simulink library "subsystems"  (R2025b)
settings: Solver=VariableStepAuto  StartTime=0.0  StopTime=10.0  RelTol=1e-3
values from neighbouring files (symbols this model uses):
  Cmdot = 1.2827224    [plant_parameters.m]
  cv = 718    [plant_parameters.m]
  g = [0 0 -9.80665]    [plant_parameters.m]
  m0 = 3.1359    [plant_parameters.m]
  T0 = 300    [plant_parameters.m]
  tank_volume = 0.009    [plant_parameters.m]
undefined symbols (not defined in the file or in its folder): DiscIntNeverNeededParam, force_controller_Ts, motor, Nozzle, platform_vel_controller, position_controller, position_controller_Ts, pressure_controller, velocity_controller, velocity_controller_Ts
libraries: simulink x14, $bdroot x6, spsFirstOrderFilterLib x2, slident x1, eeGeneralControl x1
settings Model: Creator=karadeli  LastModifiedBy=karadeli

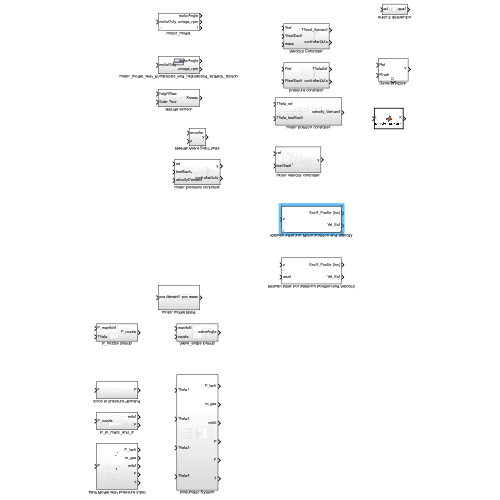
[thumbnail: Simulink's stored preview of the top-level diagram]
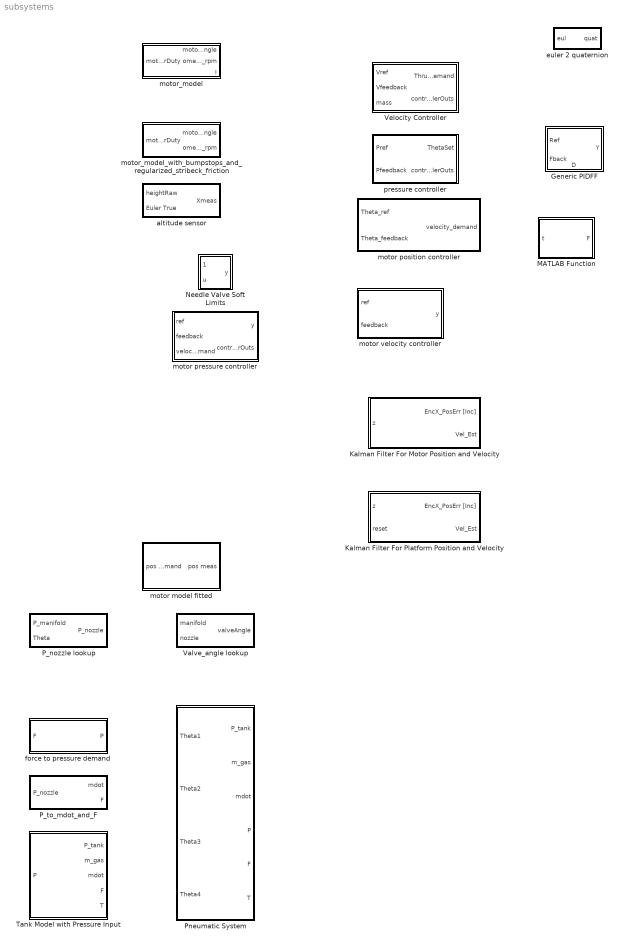
== system subsystems ==
  Generic PIDFF : Subsystem  mask{kP=0, kI=0, kD=0, kFF=0, saturation=0, saturationInt=0, rateLim=0, inputSat=0, derivativeTimeConst=0, Ts=1e-3}
      settings: PortSchema="{\"entries\":[{\"content\":{\"sides\":[{\"content\":{\"connectorIds\":[\"In1\",\"In2\"]},\"type\":\"ConnectorPlacement.EquallySpacedRectSide\",\"uuid\":\"19262ba2-78ba-44a2-8781-9b98a158f546\"},{\"content\":{\"connectorIds\":[\"Out1\"],\"side\":\"RIGHT\"},\"type\":\"ConnectorPlacement.EquallySpacedRectSide\",\"uuid\":\"f142a127-8a5f-4ee4-b1f0-7b86e0ffd133\"},{\"content\":{\"side\":\"TOP\"},\"type\":\"ConnectorPlacement.EquallySpacedRectSide\",\"uuid\":\"38fd1d3f-0c0d-4b7a-8dea-b06c7855f656\"},{\"content\":{\"connectorIds\":[\"Out2\"],\"side\":\"BOTTOM\"},\"type\":\"ConnectorPlacement.EquallySpacedRectSide\",\"uuid\":\"c6a4933e-73d5-49a0-b95d-1775e13b11db\"}]},\"type\":\"ConnectorPlacement.EquallySpacedConnector\",\"uuid\":\"e308508e-a04b-47c8-be17-ad9ebf164901\"}],\"packageUris\":[\"http://schema.mathworks.com/mf0/Connector/R2020b\"],\"version\":\"1.0\"}"
  Kalman Filter For Motor Position and Velocity : Subsystem  mask{Ts=1e-3, lambda_RQ=1}
      mask prompts: Ts "Tsample (s)"
  Kalman Filter For Platform Position and Velocity : Subsystem  mask{Ts=1e-3}
      mask prompts: Ts "Tsample (s)"
  MATLAB Function : MATLAB Function  TreatAsAtomicUnit=on
  Needle Valve Soft Limits : Subsystem
  P_nozzle lookup : Subsystem
  P_to_mdot_and_F : Subsystem
  Pneumatic System : Subsystem
  Tank Model with Pressure Input : Subsystem
  Valve_angle lookup : Subsystem
  Velocity Controller : Subsystem
  altitude sensor : Subsystem
  euler 2 quaternion : Subsystem
  force to pressure demand : Subsystem
  motor model fitted : Subsystem
  motor position controller : Subsystem
  motor pressure controller : Subsystem
  motor velocity controller : Subsystem
  motor_model : Subsystem  AncestorBlock=subsystems/motor_model_with_bumpstops_and_regularized_stribeck_friction  mask{R=6.17, Km=3.1e-2, bv=1e-4, J=1e-5, Vn=24, L=1e-6}
  motor_model_with_bumpstops_and_regularized_stribeck_friction : Subsystem
  pressure controller : Subsystem

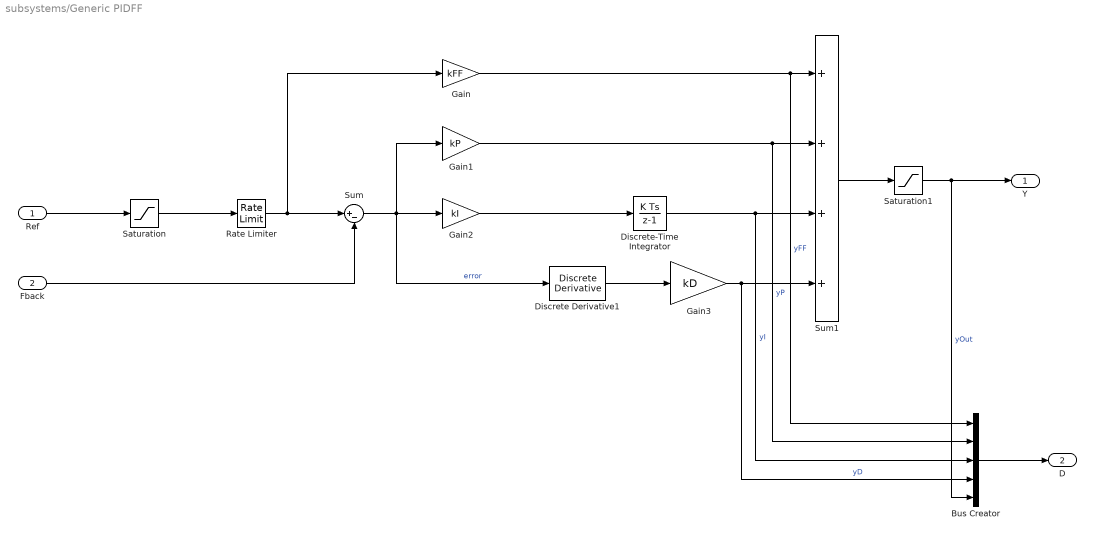
== system subsystems/Generic PIDFF ==
  Ref : Inport  PortDimensions=1  SampleTime=Ts
  Fback : Inport  Port=2  PortDimensions=1  SampleTime=Ts
  Bus Creator : BusCreator  Inputs=5
  Discrete Derivative1 : simulink/Discrete/Discrete Derivative  gainval=1.0  ICPrevScaledInput=0.0  OutMin=[]  OutMax=[]  OutDataType=fixdt(1, 16)  OutScaling=2^-10  DoSatur=off
  Discrete-Time Integrator : DiscreteIntegrator  SampleTime=Ts  LimitOutput=on  UpperSaturationLimit=saturationInt  LowerSaturationLimit=-saturationInt  ICPrevOutput=DiscIntNeverNeededParam  ICPrevScaledInput=DiscIntNeverNeededParam
  Gain : Gain  Gain=kFF
  Gain1 : Gain  Gain=kP
  Gain2 : Gain  Gain=kI
  Gain3 : Gain  Gain=kD
  Rate Limiter : RateLimiter  RisingSlewLimit=rateLim  FallingSlewLimit=-rateLim  SampleTimeMode=inherited
  Saturation : Saturate  UpperLimit=inputSat  LowerLimit=-inputSat
  Saturation1 : Saturate  UpperLimit=saturation  LowerLimit=-saturation
  Sum : Sum  Inputs=|+-
  Sum1 : Sum  Inputs=++++
  Y : Outport  PortDimensions=1  SampleTime=Ts
  D : Outport  Port=2  SampleTime=Ts
  wires:
  Bus Creator/1 -> D/1
  Discrete-Time Integrator/1 -> Sum1/3, Bus Creator/3  "yI"
  Gain1/1 -> Sum1/2, Bus Creator/2  "yP"
  Gain3/1 -> Sum1/4, Bus Creator/4  "yD"
  Saturation1/1 -> Bus Creator/5, Y/1  "yOut"
  Gain/1 -> Sum1/1, Bus Creator/1  "yFF"
  Fback/1 -> Sum/2
  Ref/1 -> Saturation/1
  Rate Limiter/1 -> Sum/1, Gain/1
  Saturation/1 -> Rate Limiter/1
  Sum/1 -> Discrete Derivative1/1, Gain2/1, Gain1/1  "error"
  Gain2/1 -> Discrete-Time Integrator/1
  Sum1/1 -> Saturation1/1
  Discrete Derivative1/1 -> Gain3/1

== system subsystems/Kalman Filter For Motor Position and Velocity ==
  z : Inport  Unit=deg  PortDimensions=1
  Resettable Delay_qk : Delay  DelayLength=1  InitialConditionSource=Input port  SampleTime=Ts
      settings: InputPortMap=u0,p4
  TPE_KALMAN_spd : MATLAB Function  TreatAsAtomicUnit=on
  Unit Delay_Pk : UnitDelay  InitialCondition=[0.155 65; 65 5.7e4]  SampleTime=Ts  HasFrameUpgradeWarning=on
  lambda_RQ : Constant  Value=lambda_RQ  OutDataTypeStr=double
  EncX_PosErr [Inc] : Outport  OutDataTypeStr=double  Unit=deg  PortDimensions=1  SampleTime=Ts  VectorParamsAs1DForOutWhenUnconnected=off
  Vel_Est : Outport  Port=2  OutDataTypeStr=double  Unit=deg/s  PortDimensions=1  SampleTime=Ts  VectorParamsAs1DForOutWhenUnconnected=off
  wires:
  Unit Delay_Pk/1 -> TPE_KALMAN_spd/4("Pk ")
  TPE_KALMAN_spd/2(posEst) -> EncX_PosErr [Inc]/1  "Pos_Est"
  Resettable Delay_qk/1 -> TPE_KALMAN_spd/3("qk ")
  TPE_KALMAN_spd/4(Pk) -> Unit Delay_Pk/1
  TPE_KALMAN_spd/3(qk) -> Resettable Delay_qk/1  "qk"
  z/1 -> Resettable Delay_qk/2, TPE_KALMAN_spd/2(z)
  lambda_RQ/1 -> TPE_KALMAN_spd/1(lambdaRQ)
  TPE_KALMAN_spd/1(velEst) -> Vel_Est/1  "Vel_Est"

== system subsystems/Kalman Filter For Platform Position and Velocity ==
  z : Inport  Unit=m  PortDimensions=1
  reset : Inport  Port=2  PortDimensions=1
  MATLAB Function : MATLAB Function  TreatAsAtomicUnit=on
  Resettable Delay_qk : Delay  DelayLength=1  InitialConditionSource=Input port  ExternalReset=Rising  SampleTime=Ts
      settings: InputPortMap=u0,r5,p4
  TPE_KALMAN_spd : MATLAB Function  TreatAsAtomicUnit=on
  Unit Delay_Pk : UnitDelay  InitialCondition=[0.155 65; 65 5.7e4]  SampleTime=Ts  HasFrameUpgradeWarning=on
  lambda_RQ : Constant  Value=2e-5  OutDataTypeStr=double
  z1 : InportShadow  Unit=m  PortDimensions=1
  EncX_PosErr [Inc] : Outport  OutDataTypeStr=double  Unit=m  PortDimensions=1  SampleTime=Ts  VectorParamsAs1DForOutWhenUnconnected=off
  Vel_Est : Outport  Port=2  OutDataTypeStr=double  Unit=m/s  PortDimensions=1  SampleTime=Ts  VectorParamsAs1DForOutWhenUnconnected=off
  wires:
  TPE_KALMAN_spd/1(velEst) -> Vel_Est/1  "Vel_Est"
  lambda_RQ/1 -> TPE_KALMAN_spd/1(lambdaRQ)
  z/1 -> TPE_KALMAN_spd/2(z)
  TPE_KALMAN_spd/3(qk) -> Resettable Delay_qk/1  "qk"
  TPE_KALMAN_spd/4(Pk) -> Unit Delay_Pk/1
  Resettable Delay_qk/1 -> TPE_KALMAN_spd/3("qk ")
  TPE_KALMAN_spd/2(posEst) -> EncX_PosErr [Inc]/1  "Pos_Est"
  Unit Delay_Pk/1 -> TPE_KALMAN_spd/4("Pk ")
  MATLAB Function/1(y) -> Resettable Delay_qk/3
  z1/1 -> MATLAB Function/1(u1)
  reset/1 -> Resettable Delay_qk/2

== system subsystems/Needle Valve Soft Limits ==
  encoder : Inport
  u : Inport  Port=2
  Constant1 : Constant  Value=-1
  Constant2 : Constant  Value=0
  Constant3 : Constant
  Constant4 : Constant  Value=0
  Saturation Dynamic : simulink/Discontinuities/Saturation Dynamic  OutMin=[]  OutMax=[]  OutDataTypeStr=Inherit: Same as second input  OutDataType=fixdt(1, 16)  OutScaling=2^-10  DoSatur=off
  Switch : Switch  Criteria=u2 > Threshold  Threshold=3*360  SaturateOnIntegerOverflow=off  InputSameDT=off
  Switch1 : Switch  Criteria=u2 > Threshold  Threshold=10  SaturateOnIntegerOverflow=off  InputSameDT=off
  y : Outport
  wires:
  Constant1/1 -> Switch1/1
  Constant4/1 -> Switch1/3
  u/1 -> Saturation Dynamic/2
  Switch1/1 -> Saturation Dynamic/3
  encoder/1 -> Switch/2, Switch1/2
  Constant3/1 -> Switch/3
  Constant2/1 -> Switch/1
  Switch/1 -> Saturation Dynamic/1
  Saturation Dynamic/1 -> y/1

== system subsystems/P_nozzle lookup ==
  P_manifold : Inport
  Theta : Inport  Port=2
  P_nozzle lookup : MATLAB Function  Commented=on  TreatAsAtomicUnit=on
  P_nozzle lookup1 : MATLAB Function  TreatAsAtomicUnit=on
  Saturation : Saturate  UpperLimit=300  LowerLimit=0
  P_nozzle : Outport
  wires:
  P_manifold/1 -> P_nozzle lookup1/1(manifold)
  Theta/1 -> P_nozzle lookup1/2(valveAngle)
  P_nozzle lookup1/1(nozzlePressure) -> Saturation/1
  Saturation/1 -> P_nozzle/1

== system subsystems/P_to_mdot_and_F ==
  P_nozzle : Inport  Unit=bar
  Gain : Gain  Gain=Nozzle.Cd
  Gain1 : Gain  Gain=1e5
  Ve1 : Gain  Gain=Nozzle.M * sqrt(1.4 * 287 / (1 + (0.2 .* Nozzle.M .* Nozzle.M)) * 300)
  kMdot3 : Gain  Gain="0.6847*pi*(Nozzle.d  * Nozzle.d)/4*1e-6/sqrt(287*300)"
  mdot : Outport  Unit=kg/s
  F : Outport  Port=2  Unit=N
  wires:
  P_nozzle/1 -> Gain1/1  "Bar"
  kMdot3/1 -> Ve1/1, mdot/1  "mdot"
  Ve1/1 -> Gain/1  "Ftheoretical"
  Gain/1 -> F/1  "Factual"
  Gain1/1 -> kMdot3/1  "Pa"

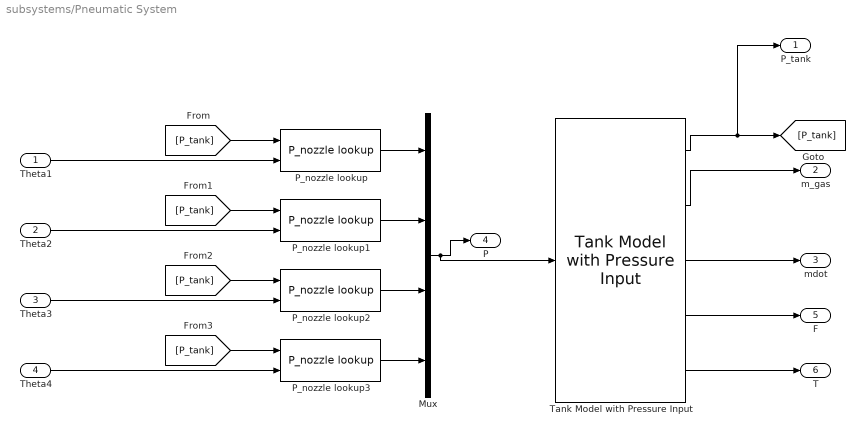
== system subsystems/Pneumatic System ==
  Theta1 : Inport
  Theta2 : Inport  Port=2
  Theta3 : Inport  Port=3
  Theta4 : Inport  Port=4
  Mux : Mux
  P_nozzle lookup{,1..3} (4 alike) : $bdroot/P_nozzle lookup  SystemSampleTime=-1  VariantActivationTime=update diagram  EmptyChoice=off  PassThrough=off  PassThroughVariantControl=(default)  EmptyChoiceVariantControl=(default)  AllowFlexibleInterface=on  Latency=0  AutoFrameSizeCalculation=off
  Tank Model with Pressure Input : $bdroot/Tank Model with Pressure Input  SystemSampleTime=-1  VariantActivationTime=update diagram  EmptyChoice=off  PassThrough=off  PassThroughVariantControl=(default)  EmptyChoiceVariantControl=(default)  AllowFlexibleInterface=on  Latency=0  AutoFrameSizeCalculation=off
  P_tank : Outport
  m_gas : Outport  Port=2
  mdot : Outport  Port=3
  P : Outport  Port=4
  F : Outport  Port=5
  T : Outport  Port=6
  wires:
  Tank Model with Pressure Input/1 -> P_tank/1, [P_tank]
  [P_tank] -> P_nozzle lookup/1
  Theta1/1 -> P_nozzle lookup/2
  Tank Model with Pressure Input/2 -> m_gas/1
  Tank Model with Pressure Input/3 -> mdot/1
  Tank Model with Pressure Input/4 -> F/1
  Tank Model with Pressure Input/5 -> T/1
  P_nozzle lookup/1 -> Mux/1
  Theta2/1 -> P_nozzle lookup1/2
  [P_tank] -> P_nozzle lookup1/1
  [P_tank] -> P_nozzle lookup3/1
  Theta4/1 -> P_nozzle lookup3/2
  Theta3/1 -> P_nozzle lookup2/2
  [P_tank] -> P_nozzle lookup2/1
  P_nozzle lookup3/1 -> Mux/4
  P_nozzle lookup2/1 -> Mux/3
  P_nozzle lookup1/1 -> Mux/2
  Mux/1 -> Tank Model with Pressure Input/1, P/1

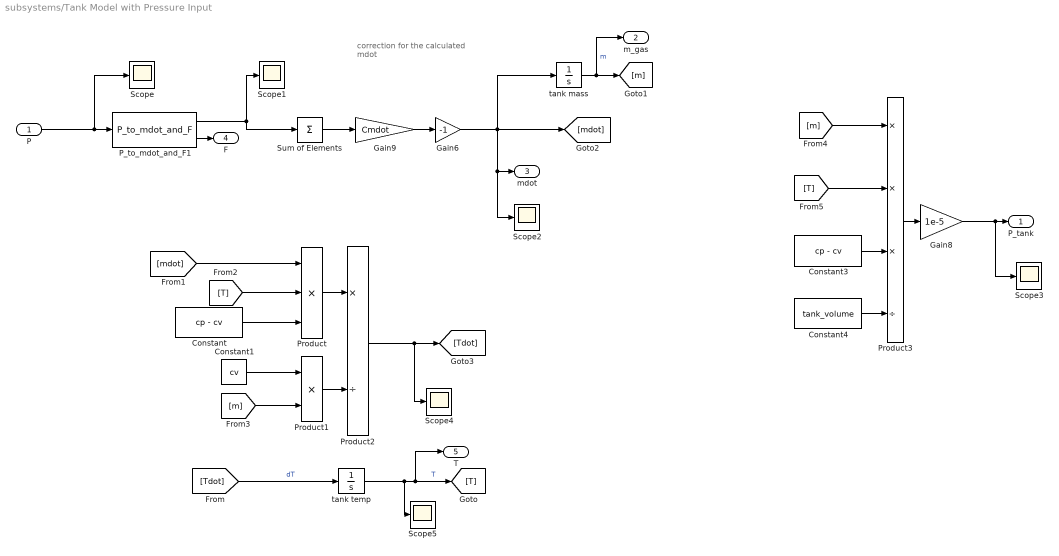
== system subsystems/Tank Model with Pressure Input ==
  note: correction for the calculated mdot
  P : Inport
  Constant : Constant  Value=cp - cv
  Constant1 : Constant  Value=cv
  Constant3 : Constant  Value=cp - cv
  Constant4 : Constant  Value=tank_volume
  Gain6 : Gain  Gain=-1
  Gain8 : Gain  Gain=1e-5
  Gain9 : Gain  Gain=Cmdot
  P_to_mdot_and_F1 : $bdroot/P_to_mdot_and_F  SystemSampleTime=-1  VariantActivationTime=update diagram  AllowFlexibleInterface=on  Latency=0  AutoFrameSizeCalculation=off
  Product : Product  Inputs=3
  Product1 : Product
  Product2 : Product  Inputs=*/
  Product3 : Product  Inputs=***/
  Scope{,1..5} (6 alike) : Scope
      Scope1 settings: DataLoggingVariableName=ScopeData2
      Scope2 settings: DataLoggingVariableName=ScopeData3
      Scope3 settings: DataLoggingVariableName=ScopeData4
      Scope4 settings: DataLoggingVariableName=ScopeData5
      Scope5 settings: DataLoggingVariableName=ScopeData6
  Sum of Elements : Sum  Inputs=+
  tank mass : Integrator  InitialCondition=m0  LimitOutput=on  LowerSaturationLimit=0
  tank temp : Integrator  InitialCondition=T0
  P_tank : Outport
  m_gas : Outport  Port=2
  mdot : Outport  Port=3
  F : Outport  Port=4
  T : Outport  Port=5
  wires:
  Constant3/1 -> Product3/3
  [T] -> Product/2
  tank mass/1 -> m_gas/1, [m]  "m"
  Gain9/1 -> Gain6/1
  [m] -> Product3/1
  Sum of Elements/1 -> Gain9/1
  [Tdot] -> tank temp/1  "dT"
  Product3/1 -> Gain8/1
  Gain6/1 -> tank mass/1, Scope2/1, mdot/1, [mdot]
  Product/1 -> Product2/1
  [m] -> Product1/2
  Constant/1 -> Product/3
  Product1/1 -> Product2/2
  Constant1/1 -> Product1/1
  P/1 -> Scope/1, P_to_mdot_and_F1/1
  tank temp/1 -> Scope5/1, T/1, [T]  "T"
  [T] -> Product3/2
  [mdot] -> Product/1
  Constant4/1 -> Product3/4
  Gain8/1 -> Scope3/1, P_tank/1
  Product2/1 -> Scope4/1, [Tdot]
  P_to_mdot_and_F1/2 -> F/1
  P_to_mdot_and_F1/1 -> Scope1/1, Sum of Elements/1

== system subsystems/Valve_angle lookup ==
  manifold : Inport
  nozzle : Inport  Port=2
  Constant : Constant  Value=150
  P_nozzle lookup : MATLAB Function  Commented=on  TreatAsAtomicUnit=on
  P_nozzle lookup1 : MATLAB Function  TreatAsAtomicUnit=on
  Saturation : Saturate  UpperLimit=3*360  LowerLimit=0
  valveAngle : Outport
  wires:
  P_nozzle lookup1/1(valveAngle) -> Saturation/1
  manifold/1 -> P_nozzle lookup1/1(manifold)
  nozzle/1 -> P_nozzle lookup1/2(nozzle)
  Saturation/1 -> valveAngle/1
  Constant/1 -> P_nozzle lookup1/3(angle0)

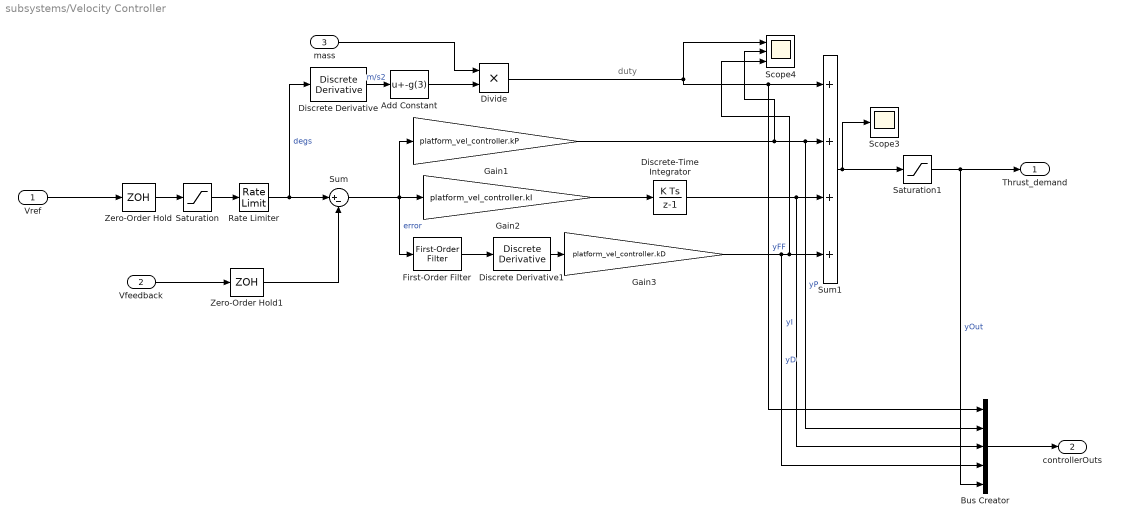
== system subsystems/Velocity Controller ==
  note: duty
  Vref : Inport  Unit=m/s  PortDimensions=1
  Vfeedback : Inport  Port=2  Unit=m/s  PortDimensions=1
  mass : Inport  Port=3  Unit=kg  PortDimensions=1
  Add Constant : Bias  Bias=-g(3)  SaturateOnIntegerOverflow=off
  Bus Creator : BusCreator  Inputs=5
  Discrete Derivative : simulink/Discrete/Discrete Derivative  gainval=1.0  ICPrevScaledInput=0.0  OutMin=[]  OutMax=[]  OutDataType=fixdt(1, 16)  OutScaling=2^-10  DoSatur=off
  Discrete Derivative1 : simulink/Discrete/Discrete Derivative  gainval=1.0  ICPrevScaledInput=0.0  OutMin=[]  OutMax=[]  OutDataType=fixdt(1, 16)  OutScaling=2^-10  DoSatur=off
  Discrete-Time Integrator : DiscreteIntegrator  SampleTime=-1  LimitOutput=on  UpperSaturationLimit=platform_vel_controller.saturationInt  LowerSaturationLimit=-platform_vel_controller.saturationInt  ICPrevOutput=DiscIntNeverNeededParam  ICPrevScaledInput=DiscIntNeverNeededParam
  Divide : Product  Inputs=**
  First-Order Filter : spsFirstOrderFilterLib/First-Order Filter  FilterType=Lowpass  Tc=10e-3  Ts=1e-3  Initialize=on  Vac_Init=[0, 0, 60]  Vdc_Init=0  PlotResponse=off  FreqRange="[0,  200,  1]"
  Gain1 : Gain  Gain=platform_vel_controller.kP
  Gain2 : Gain  Gain=platform_vel_controller.kI
  Gain3 : Gain  Gain=platform_vel_controller.kD
  Rate Limiter : RateLimiter  RisingSlewLimit=platform_vel_controller.rateLimiter  FallingSlewLimit=-platform_vel_controller.rateLimiter  SampleTimeMode=inherited
  Saturation : Saturate  UpperLimit=480/60*360  LowerLimit=-480/60*360
  Saturation1 : Saturate  UpperLimit=platform_vel_controller.saturation  LowerLimit=-platform_vel_controller.saturation
  Scope3 : Scope
      settings: ActiveDisplayYMinimum=-1.71173  ActiveDisplayYMaximum=1.27546  DataLoggingVariableName=ScopeData5
  Scope4 : Scope  NumInputPorts=3
      settings: ActiveDisplayYMinimum=-1.04128  ActiveDisplayYMaximum=0.98598  DataLoggingVariableName=ScopeData11
  Sum : Sum  Inputs=|+-
  Sum1 : Sum  Inputs=++++
  Zero-Order Hold : ZeroOrderHold  SampleTime=1e-3
  Zero-Order Hold1 : ZeroOrderHold  SampleTime=1e-3
  Thrust_demand : Outport  Unit=N  PortDimensions=1
  controllerOuts : Outport  Port=2
  wires:
  Bus Creator/1 -> controllerOuts/1
  Discrete-Time Integrator/1 -> Sum1/3, Bus Creator/3  "yI"
  Gain1/1 -> Scope4/2, Sum1/2, Bus Creator/2  "yP"
  Gain3/1 -> Scope4/3, Sum1/4, Bus Creator/4  "yD"
  Saturation1/1 -> Bus Creator/5, Thrust_demand/1  "yOut"
  Divide/1 -> Sum1/1, Bus Creator/1, Scope4/1  "yFF"
  Zero-Order Hold1/1 -> Sum/2
  Vfeedback/1 -> Zero-Order Hold1/1
  Zero-Order Hold/1 -> Saturation/1
  Vref/1 -> Zero-Order Hold/1
  Rate Limiter/1 -> Sum/1, Discrete Derivative/1  "degs"
  Saturation/1 -> Rate Limiter/1
  Sum/1 -> First-Order Filter/1, Gain1/1, Gain2/1  "error"
  Gain2/1 -> Discrete-Time Integrator/1
  Sum1/1 -> Scope3/1, Saturation1/1
  Discrete Derivative1/1 -> Gain3/1
  First-Order Filter/1 -> Discrete Derivative1/1
  Discrete Derivative/1 -> Add Constant/1  "m/s2"
  Add Constant/1 -> Divide/2
  mass/1 -> Divide/1

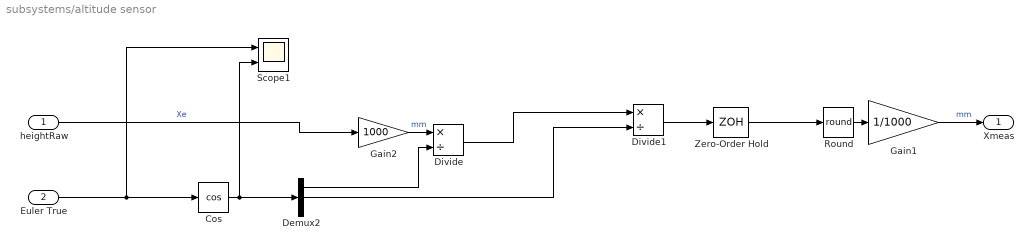
== system subsystems/altitude sensor ==
  heightRaw : Inport
  Euler True : Inport  Port=2
  Cos : Trigonometry  Operator=cos
  Demux2 : Demux  Outputs=3
  Divide : Product  Inputs=*/
  Divide1 : Product  Inputs=*/
  Gain1 : Gain  Gain=1/1000
  Gain2 : Gain  Gain=1000
  Round : Rounding  Operator=round
  Scope1 : Scope  NumInputPorts=2
      settings: ActiveDisplayYMinimum=-0.45593  ActiveDisplayYMaximum=1.16177
  Zero-Order Hold : ZeroOrderHold  SampleTime=1/1000
  Xmeas : Outport
  wires:
  Euler True/1 -> Cos/1, Scope1/1
  Cos/1 -> Demux2/1, Scope1/2
  Round/1 -> Gain1/1
  Demux2/2 -> Divide1/2
  Demux2/1 -> Divide/2
  Gain2/1 -> Divide/1  "mm"
  Divide/1 -> Divide1/1
  Zero-Order Hold/1 -> Round/1
  heightRaw/1 -> Gain2/1  "Xe"
  Divide1/1 -> Zero-Order Hold/1
  Gain1/1 -> Xmeas/1  "mm"

== system subsystems/euler 2 quaternion ==
  eul : Inport  PortDimensions=3
  Demux : Demux  Outputs=3
  MATLAB Function : MATLAB Function  TreatAsAtomicUnit=on
  Mux : Mux
  quat : Outport  PortDimensions=4
  wires:
  Demux/2 -> MATLAB Function/2(u2)
  Demux/3 -> MATLAB Function/3(u3)
  eul/1 -> Demux/1
  Demux/1 -> MATLAB Function/1(u1)
  MATLAB Function/2(y2) -> Mux/2
  MATLAB Function/3(y3) -> Mux/3
  MATLAB Function/4(y4) -> Mux/4
  MATLAB Function/1(y1) -> Mux/1
  Mux/1 -> quat/1

== system subsystems/force to pressure demand ==
  F : Inport  Unit=N  SampleTime=force_controller_Ts
  Gain2 : Gain  Gain=1./Nozzle.Cd
  Gain3 : Gain  Gain=1e-5
  Ve2 : Gain  Gain=1/(Nozzle.M * sqrt(1.4 * 287 / (1 + (0.2 * Nozzle.M*Nozzle.M)) * 300))
  kMdot1 : Gain  Gain=1/(0.6847*pi*(Nozzle.d*Nozzle.d)/4*1e-6/sqrt(287*300))
  P : Outport  Unit=bar  SampleTime=force_controller_Ts
  wires:
  F/1 -> Gain2/1
  Gain2/1 -> Ve2/1  "Ftheo"
  Ve2/1 -> kMdot1/1  "Mdot"
  kMdot1/1 -> Gain3/1  "Pa"
  Gain3/1 -> P/1  "Bar"

== system subsystems/motor model fitted ==
  pos demand : Inport
  Rate Limiter : RateLimiter  RisingSlewLimit=position_controller.rateLimiter  FallingSlewLimit=-position_controller.rateLimiter  SampleTimeMode=inherited
  Saturation : Saturate  UpperLimit=4*360  LowerLimit=-10
  motor model fitted : slident/Models/Idmodel  sys=ss3  IC=0  noi=off  seed=[]
  pos meas : Outport
  wires:
  motor model fitted/1 -> pos meas/1
  pos demand/1 -> Saturation/1
  Saturation/1 -> Rate Limiter/1
  Rate Limiter/1 -> motor model fitted/1  "degs"

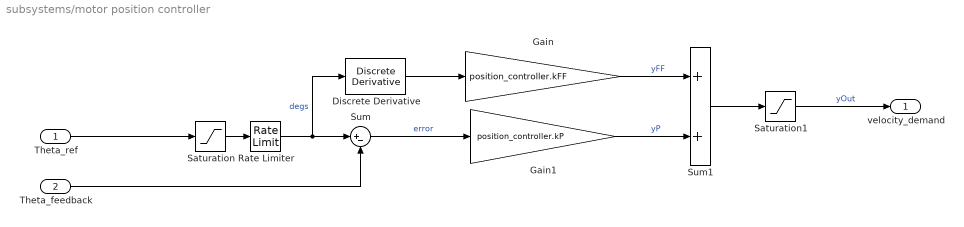
== system subsystems/motor position controller ==
  Theta_ref : Inport  Unit=deg  SampleTime=position_controller_Ts
  Theta_feedback : Inport  Port=2  Unit=deg  SampleTime=position_controller_Ts
  Discrete Derivative : simulink/Discrete/Discrete Derivative  gainval=1.0  ICPrevScaledInput=0.0  OutMin=[]  OutMax=[]  OutDataType=fixdt(1, 16)  OutScaling=2^-10  DoSatur=off
  Gain : Gain  Gain=position_controller.kFF
  Gain1 : Gain  Gain=position_controller.kP
  Rate Limiter : RateLimiter  RisingSlewLimit=position_controller.rateLimiter  FallingSlewLimit=-position_controller.rateLimiter  SampleTimeMode=inherited
  Saturation : Saturate  UpperLimit=4*360  LowerLimit=-10
  Saturation1 : Saturate  UpperLimit=position_controller.saturation  LowerLimit=-position_controller.saturation
  Sum : Sum  Inputs=|+-
  Sum1 : Sum
  velocity_demand : Outport  Unit=deg/s  SampleTime=position_controller_Ts
  wires:
  Sum1/1 -> Saturation1/1
  Sum/1 -> Gain1/1  "error"
  Saturation/1 -> Rate Limiter/1
  Rate Limiter/1 -> Sum/1, Discrete Derivative/1  "degs"
  Theta_ref/1 -> Saturation/1
  Theta_feedback/1 -> Sum/2
  Saturation1/1 -> velocity_demand/1  "yOut"
  Gain1/1 -> Sum1/2  "yP"
  Gain/1 -> Sum1/1  "yFF"
  Discrete Derivative/1 -> Gain/1

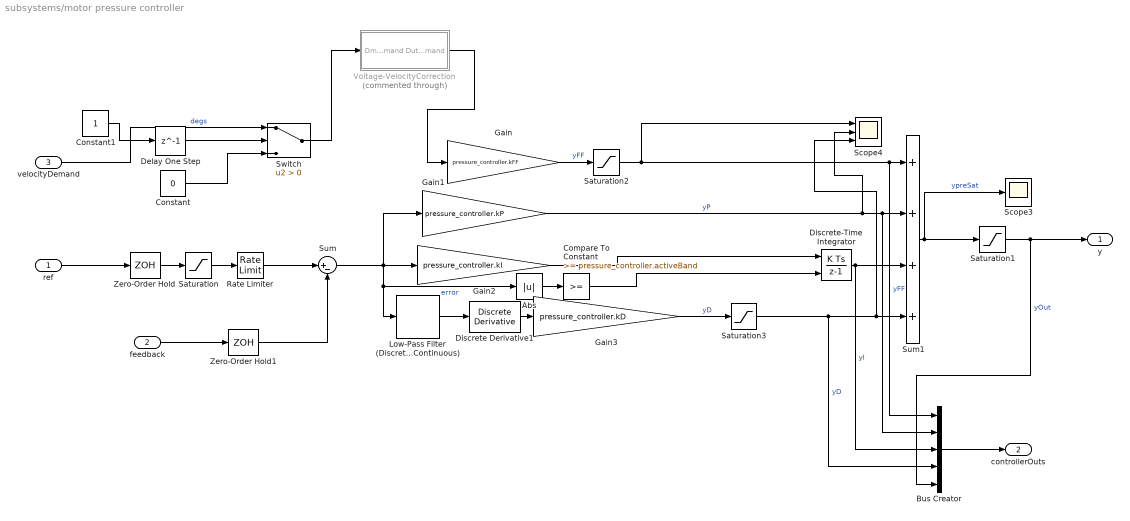
== system subsystems/motor pressure controller ==
  ref : Inport
  feedback : Inport  Port=2
  velocityDemand : Inport  Port=3
  Abs : Abs  SaturateOnIntegerOverflow=off
  Bus Creator : BusCreator  Inputs=5
  Compare To Constant : simulink/Logic and Bit Operations/Compare To Constant  relop=>=  const=pressure_controller.activeBand  OutDataTypeStr=boolean
  Constant : Constant  Value=0
  Constant1 : Constant
  Delay One Step : Delay  DelayLength=1  SampleTime=1e-3
  Discrete Derivative1 : simulink/Discrete/Discrete Derivative  gainval=1.0  ICPrevScaledInput=0.0  OutMin=[]  OutMax=[]  OutDataType=fixdt(1, 16)  OutScaling=2^-10  DoSatur=off
  Discrete-Time Integrator : DiscreteIntegrator  ExternalReset=level  SampleTime=1e-3  LimitOutput=on  UpperSaturationLimit=pressure_controller.integralSaturation  LowerSaturationLimit=-pressure_controller.integralSaturation  ICPrevOutput=DiscIntNeverNeededParam  ICPrevScaledInput=DiscIntNeverNeededParam
  Gain : Gain  Gain=pressure_controller.kFF
  Gain1 : Gain  Gain=pressure_controller.kP
  Gain2 : Gain  Gain=pressure_controller.kI
  Gain3 : Gain  Gain=pressure_controller.kD
  Low-Pass Filter (Discrete or Continuous) : eeGeneralControl/Low-Pass Filter (Discrete or Continuous)  K=1  T=10e-3  B=1e5  A=-1e5  init_option=Inherited from block input  x0=0  Ts=1e-3
  Rate Limiter : RateLimiter  RisingSlewLimit=pressure_controller.rateLimiter  FallingSlewLimit=-pressure_controller.rateLimiter  SampleTimeMode=inherited
  Saturation : Saturate  UpperLimit=250  LowerLimit=0
  Saturation1 : Saturate  UpperLimit=1  LowerLimit=-1
  Saturation2 : Saturate  UpperLimit=1  LowerLimit=-1
  Saturation3 : Saturate  UpperLimit=1  LowerLimit=-1
  Scope3 : Scope
      settings: ActiveDisplayYMinimum=-1.71173  ActiveDisplayYMaximum=1.27546  DataLoggingVariableName=ScopeData5
  Scope4 : Scope  NumInputPorts=3
      settings: ActiveDisplayYMinimum=-1.04128  ActiveDisplayYMaximum=0.98598  DataLoggingVariableName=ScopeData11
  Sum : Sum  Inputs=|+-
  Sum1 : Sum  Inputs=++++
  Switch : Switch  Criteria=u2 > Threshold  SaturateOnIntegerOverflow=off  InputSameDT=off
  Voltage-VelocityCorrection : Subsystem  Commented=through
  Zero-Order Hold : ZeroOrderHold  SampleTime=1e-3
  Zero-Order Hold1 : ZeroOrderHold  SampleTime=1e-3
  y : Outport
  controllerOuts : Outport  Port=2
  wires:
  Zero-Order Hold1/1 -> Sum/2
  feedback/1 -> Zero-Order Hold1/1
  Zero-Order Hold/1 -> Saturation/1
  Gain/1 -> Saturation2/1  "yFF"
  ref/1 -> Zero-Order Hold/1
  velocityDemand/1 -> Switch/1  "degs"
  Saturation/1 -> Rate Limiter/1
  Sum/1 -> Gain1/1, Gain2/1, Abs/1, Low-Pass Filter (Discrete or Continuous)/1  "error"
  Gain2/1 -> Discrete-Time Integrator/1
  Sum1/1 -> Scope3/1, Saturation1/1  "ypreSat"
  Saturation1/1 -> Bus Creator/5, y/1  "yOut"
  Rate Limiter/1 -> Sum/1
  Discrete Derivative1/1 -> Gain3/1
  Gain1/1 -> Scope4/2, Bus Creator/2, Sum1/2  "yP"
  Low-Pass Filter (Discrete or Continuous)/1 -> Discrete Derivative1/1
  Gain3/1 -> Saturation3/1  "yD"
  Abs/1 -> Compare To Constant/1
  Compare To Constant/1 -> Discrete-Time Integrator/2
  Discrete-Time Integrator/1 -> Bus Creator/3, Sum1/3  "yI"
  Bus Creator/1 -> controllerOuts/1
  Saturation2/1 -> Scope4/1, Bus Creator/1, Sum1/1  "yFF"
  Switch/1 -> Voltage-VelocityCorrection/1(OmegaDemand)
  Delay One Step/1 -> Switch/2
  Constant/1 -> Switch/3
  Constant1/1 -> Delay One Step/1
  Saturation3/1 -> Bus Creator/4, Scope4/3, Sum1/4  "yD"
  Voltage-VelocityCorrection/1(DutyDemand) -> Gain/1

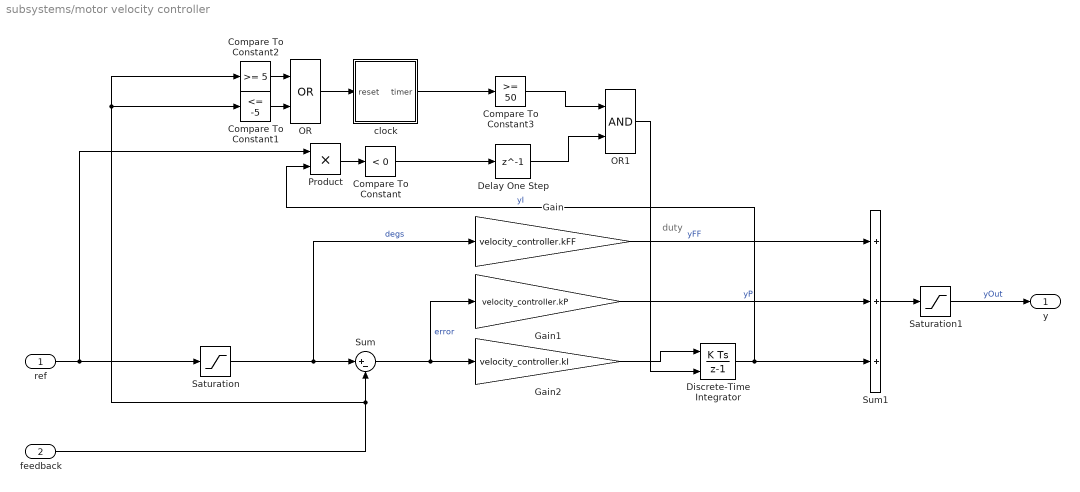
== system subsystems/motor velocity controller ==
  note: duty
  ref : Inport  SampleTime=velocity_controller_Ts
  feedback : Inport  Port=2  SampleTime=velocity_controller_Ts
  Compare To Constant : simulink/Logic and Bit Operations/Compare To Constant  relop=<  const=0  OutDataTypeStr=boolean
  Compare To Constant1 : simulink/Logic and Bit Operations/Compare To Constant  relop=<=  const=-5  OutDataTypeStr=boolean
  Compare To Constant2 : simulink/Logic and Bit Operations/Compare To Constant  relop=>=  const=5  OutDataTypeStr=boolean
  Compare To Constant3 : simulink/Logic and Bit Operations/Compare To Constant  relop=>=  const=50  OutDataTypeStr=boolean
  Delay One Step : Delay  DelayLength=1  SampleTime=velocity_controller_Ts
  Discrete-Time Integrator : DiscreteIntegrator  ExternalReset=rising  SampleTime=-1  LimitOutput=on  UpperSaturationLimit=1  LowerSaturationLimit=-1  ICPrevOutput=DiscIntNeverNeededParam  ICPrevScaledInput=DiscIntNeverNeededParam
  Gain : Gain  Gain=velocity_controller.kFF
  Gain1 : Gain  Gain=velocity_controller.kP
  Gain2 : Gain  Gain=velocity_controller.kI
  OR : Logic  Operator=OR  IconShape=distinctive  AllPortsSameDT=off  OutDataTypeStr=boolean
  OR1 : Logic  AllPortsSameDT=off  OutDataTypeStr=boolean
  Product : Product
  Saturation : Saturate  UpperLimit=480/60*360  LowerLimit=-480/60*360
  Saturation1 : Saturate  UpperLimit=1  LowerLimit=-1
  Sum : Sum  Inputs=|+-
  Sum1 : Sum  Inputs=+++
  clock : Subsystem
  y : Outport  SampleTime=velocity_controller_Ts
  wires:
  Discrete-Time Integrator/1 -> Product/2, Sum1/3  "yI"
  Gain1/1 -> Sum1/2  "yP"
  Saturation1/1 -> y/1  "yOut"
  Gain/1 -> Sum1/1  "yFF"
  feedback/1 -> Compare To Constant2/1, Compare To Constant1/1, Sum/2
  ref/1 -> Saturation/1, Product/1
  Saturation/1 -> Sum/1, Gain/1  "degs"
  Sum/1 -> Gain1/1, Gain2/1  "error"
  Gain2/1 -> Discrete-Time Integrator/1
  Sum1/1 -> Saturation1/1
  OR/1 -> clock/1(reset)
  clock/1(timer) -> Compare To Constant3/1
  Compare To Constant1/1 -> OR/2
  Compare To Constant2/1 -> OR/1
  Product/1 -> Compare To Constant/1
  Compare To Constant3/1 -> OR1/1
  Compare To Constant/1 -> Delay One Step/1
  OR1/1 -> Discrete-Time Integrator/2
  Delay One Step/1 -> OR1/2

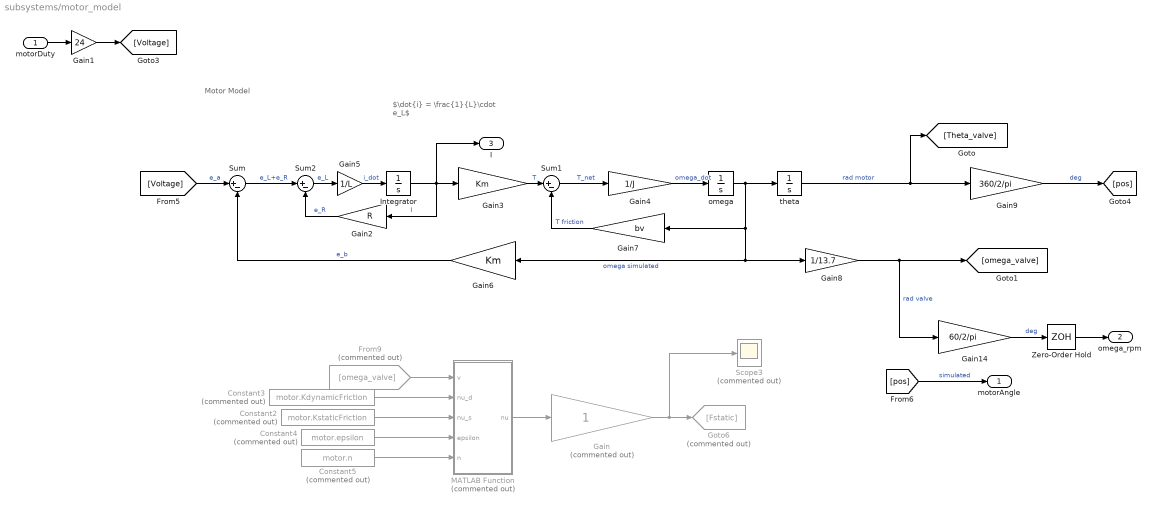
== system subsystems/motor_model ==
  note: $\dot{i} = \frac{1}{L}\cdot e_L$
  note: Motor Model
  motorDuty : Inport  PortDimensions=1
  Constant2 : Constant  Commented=on  Value=motor.KstaticFriction
  Constant3 : Constant  Commented=on  Value=motor.KdynamicFriction
  Constant4 : Constant  Commented=on  Value=motor.epsilon
  Constant5 : Constant  Commented=on  Value=motor.n
  From9 : From  Commented=on  GotoTag=omega_valve
  Gain : Gain  Commented=on
  Gain1 : Gain  Gain=24
  Gain14 : Gain  Gain=60/2/pi
  Gain2 : Gain  Gain=R
  Gain3 : Gain  Gain=Km
  Gain4 : Gain  Gain=1/J
  Gain5 : Gain  Gain=1/L
  Gain6 : Gain  Gain=Km
  Gain7 : Gain  Gain=bv
  Gain8 : Gain  Gain=1/13.7
  Gain9 : Gain  Gain=360/2/pi
  Goto6 : Goto  Commented=on  GotoTag=Fstatic
  Integrator : Integrator
  MATLAB Function : MATLAB Function  Commented=on  TreatAsAtomicUnit=on
  Scope3 : Scope  Commented=on
      settings: ActiveDisplayYMinimum=-5132.32651  ActiveDisplayYMaximum=2204.97475
  Sum : Sum  Inputs=|+-
  Sum1 : Sum  Inputs=|+-
  Sum2 : Sum  Inputs=|+-
  Zero-Order Hold : ZeroOrderHold  SampleTime=1e-3
  omega : Integrator
  theta : Integrator  ZeroCross=off
  motorAngle : Outport  Unit=1
  omega_rpm : Outport  Port=2
  I : Outport  Port=3  Unit=A
  wires:
  Gain1/1 -> [Voltage]
  Sum2/1 -> Gain5/1  "e_L"
  MATLAB Function/1(nu) -> Gain/1
  Gain14/1 -> Zero-Order Hold/1  "deg"
  omega/1 -> theta/1, Gain7/1, Gain8/1, Gain6/1  "omega simulated"
  Gain9/1 -> [pos]  "deg"
  [Voltage] -> Sum/1  "e_a"
  Gain4/1 -> omega/1  "omega_dot"
  Gain8/1 -> Gain14/1, [omega_valve]  "rad valve"
  Sum1/1 -> Gain4/1  "T_net"
  Sum/1 -> Sum2/1  "e_L+e_R"
  Gain7/1 -> Sum1/2  "T friction"
  From9/1 -> MATLAB Function/1(v)
  Constant4/1 -> MATLAB Function/4(epsilon)
  motorDuty/1 -> Gain1/1
  Gain/1 -> Scope3/1, Goto6/1
  Zero-Order Hold/1 -> omega_rpm/1
  Constant5/1 -> MATLAB Function/5(n)
  Gain6/1 -> Sum/2  "e_b"
  Gain3/1 -> Sum1/1  "T"
  theta/1 -> [Theta_valve], Gain9/1  "rad motor"
  Constant3/1 -> MATLAB Function/2(nu_d)
  Constant2/1 -> MATLAB Function/3(nu_s)
  [pos] -> motorAngle/1  "simulated"
  Integrator/1 -> Gain2/1, I/1, Gain3/1  "I"
  Gain2/1 -> Sum2/2  "e_R"
  Gain5/1 -> Integrator/1  "i_dot"

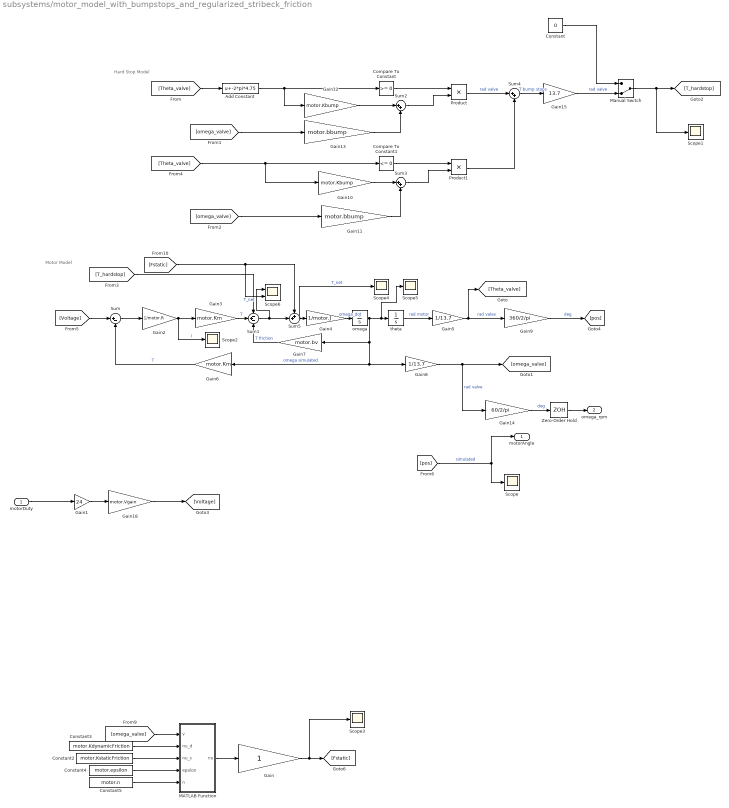
== system subsystems/motor_model_with_bumpstops_and_regularized_stribeck_friction ==
  note: Hard Stop Model
  note: Motor Model
  motorDuty : Inport  PortDimensions=1
  Add Constant : Bias  Bias=-2*pi*4.75  SaturateOnIntegerOverflow=off
  Compare To Constant : simulink/Logic and Bit Operations/Compare To Constant  relop=>=  const=0  OutDataTypeStr=boolean
  Compare To Constant1 : simulink/Logic and Bit Operations/Compare To Constant  relop=<=  const=0  OutDataTypeStr=boolean
  Constant : Constant  Value=0
  Constant2 : Constant  Value=motor.KstaticFriction
  Constant3 : Constant  Value=motor.KdynamicFriction
  Constant4 : Constant  Value=motor.epsilon
  Constant5 : Constant  Value=motor.n
  Gain : Gain
  Gain1 : Gain  Gain=24
  Gain10 : Gain  Gain=motor.Kbump
  Gain11 : Gain  Gain=motor.bbump
  Gain12 : Gain  Gain=motor.Kbump
  Gain13 : Gain  Gain=motor.bbump
  Gain14 : Gain  Gain=60/2/pi
  Gain15 : Gain  Gain=13.7
  Gain18 : Gain  Gain=motor.Vgain
  Gain2 : Gain  Gain=1/motor.R
  Gain3 : Gain  Gain=motor.Km
  Gain4 : Gain  Gain=1/motor.J
  Gain5 : Gain  Gain=1/13.7
  Gain6 : Gain  Gain=motor.Km
  Gain7 : Gain  Gain=motor.bv
  Gain8 : Gain  Gain=1/13.7
  Gain9 : Gain  Gain=360/2/pi
  MATLAB Function : MATLAB Function  TreatAsAtomicUnit=on
  Manual Switch : ManualSwitch  CurrentSetting=0
  Product : Product
  Product1 : Product
  Scope{,1..5} (6 alike) : Scope
      Scope settings: ActiveDisplayYMinimum=-5132.32651  ActiveDisplayYMaximum=2204.97475
      Scope2 settings: ActiveDisplayYMinimum=-6.0528  ActiveDisplayYMaximum=4.68117  DataLoggingVariableName=ScopeData3
      Scope3 settings: ActiveDisplayYMinimum=-5132.32651  ActiveDisplayYMaximum=2204.97475
  Scope6 : Scope  NumInputPorts=2
  Sum : Sum  Inputs=|+-
  Sum1 : Sum  Inputs=-+-
  Sum2 : Sum  Inputs=|++
  Sum3 : Sum  Inputs=|++
  Sum4 : Sum  Inputs=|++
  Sum5 : Sum  Inputs=++|
  Zero-Order Hold : ZeroOrderHold  SampleTime=1e-3
  omega : Integrator
  theta : Integrator  ZeroCross=off
  motorAngle : Outport  Unit=1
  omega_rpm : Outport  Port=2
  wires:
  [pos] -> motorAngle/1, Scope/1  "simulated"
  Constant2/1 -> MATLAB Function/3(nu_s)
  Constant3/1 -> MATLAB Function/2(nu_d)
  Gain15/1 -> Manual Switch/2  "rad valve"
  [Fstatic] -> Scope6/2, Sum5/1
  theta/1 -> Gain5/1  "rad motor"
  Product1/1 -> Sum4/2
  Gain3/1 -> Sum1/2  "T"
  Gain6/1 -> Sum/2  "T"
  Sum2/1 -> Product/2
  Gain10/1 -> Sum3/1
  Add Constant/1 -> Gain12/1, Compare To Constant/1
  Gain12/1 -> Sum2/1
  Product/1 -> Sum4/1  "rad valve"
  Constant5/1 -> MATLAB Function/5(n)
  Gain11/1 -> Sum3/2
  Zero-Order Hold/1 -> omega_rpm/1
  [omega_valve] -> Gain11/1
  Sum3/1 -> Product1/2
  Gain/1 -> [Fstatic], Scope3/1
  Gain13/1 -> Sum2/2
  Manual Switch/1 -> [T_hardstop], Scope1/1
  motorDuty/1 -> Gain1/1
  Constant4/1 -> MATLAB Function/4(epsilon)
  [T_hardstop] -> Sum1/1
  [omega_valve] -> MATLAB Function/1(v)
  Gain7/1 -> Sum1/3  "T friction"
  Sum/1 -> Gain2/1
  Sum5/1 -> Gain4/1, Scope4/1  "T_net"
  Sum1/1 -> Sum5/2, Scope6/1  "T_net"
  Sum4/1 -> Gain15/1  "T bump stops"
  Compare To Constant1/1 -> Product1/1
  Gain8/1 -> [omega_valve], Gain14/1  "rad valve"
  Gain4/1 -> omega/1  "omega_dot"
  Compare To Constant/1 -> Product/1
  [Voltage] -> Sum/1
  [Theta_valve] -> Gain10/1, Compare To Constant1/1
  Gain9/1 -> [pos]  "deg"
  Gain5/1 -> Gain9/1, [Theta_valve]  "rad valve"
  omega/1 -> Gain6/1, Gain8/1, Gain7/1, theta/1, Scope5/1  "omega simulated"
  Gain14/1 -> Zero-Order Hold/1  "deg"
  MATLAB Function/1(nu) -> Gain/1
  Gain1/1 -> Gain18/1
  [omega_valve] -> Gain13/1
  Gain2/1 -> Scope2/1, Gain3/1  "I"
  Constant/1 -> Manual Switch/1
  [Theta_valve] -> Add Constant/1
  Gain18/1 -> [Voltage]

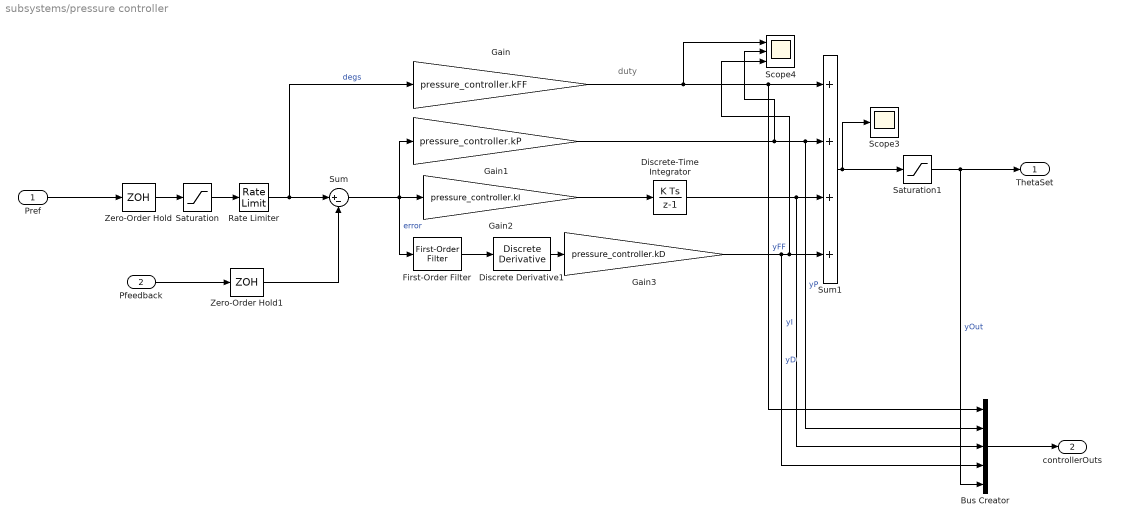
== system subsystems/pressure controller ==
  note: duty
  Pref : Inport
  Pfeedback : Inport  Port=2
  Bus Creator : BusCreator  Inputs=5
  Discrete Derivative1 : simulink/Discrete/Discrete Derivative  gainval=1.0  ICPrevScaledInput=0.0  OutMin=[]  OutMax=[]  OutDataType=fixdt(1, 16)  OutScaling=2^-10  DoSatur=off
  Discrete-Time Integrator : DiscreteIntegrator  SampleTime=-1  LimitOutput=on  UpperSaturationLimit=1  LowerSaturationLimit=-1  ICPrevOutput=DiscIntNeverNeededParam  ICPrevScaledInput=DiscIntNeverNeededParam
  First-Order Filter : spsFirstOrderFilterLib/First-Order Filter  FilterType=Lowpass  Tc=10e-3  Ts=1e-3  Initialize=on  Vac_Init=[0, 0, 60]  Vdc_Init=0  PlotResponse=off  FreqRange="[0,  200,  1]"
  Gain : Gain  Gain=pressure_controller.kFF
  Gain1 : Gain  Gain=pressure_controller.kP
  Gain2 : Gain  Gain=pressure_controller.kI
  Gain3 : Gain  Gain=pressure_controller.kD
  Rate Limiter : RateLimiter  RisingSlewLimit=1e15  FallingSlewLimit=-1e15  SampleTimeMode=inherited
  Saturation : Saturate  UpperLimit=480/60*360  LowerLimit=-480/60*360
  Saturation1 : Saturate  UpperLimit=1  LowerLimit=-1
  Scope3 : Scope
      settings: ActiveDisplayYMinimum=-1.71173  ActiveDisplayYMaximum=1.27546  DataLoggingVariableName=ScopeData5
  Scope4 : Scope  NumInputPorts=3
      settings: ActiveDisplayYMinimum=-1.04128  ActiveDisplayYMaximum=0.98598  DataLoggingVariableName=ScopeData11
  Sum : Sum  Inputs=|+-
  Sum1 : Sum  Inputs=++++
  Zero-Order Hold : ZeroOrderHold  SampleTime=1e-3
  Zero-Order Hold1 : ZeroOrderHold  SampleTime=1e-3
  ThetaSet : Outport
  controllerOuts : Outport  Port=2
  wires:
  First-Order Filter/1 -> Discrete Derivative1/1
  Discrete Derivative1/1 -> Gain3/1
  Sum1/1 -> Saturation1/1, Scope3/1
  Gain2/1 -> Discrete-Time Integrator/1
  Sum/1 -> Gain2/1, Gain1/1, First-Order Filter/1  "error"
  Saturation/1 -> Rate Limiter/1
  Rate Limiter/1 -> Gain/1, Sum/1  "degs"
  Pref/1 -> Zero-Order Hold/1
  Zero-Order Hold/1 -> Saturation/1
  Pfeedback/1 -> Zero-Order Hold1/1
  Zero-Order Hold1/1 -> Sum/2
  Gain/1 -> Bus Creator/1, Sum1/1, Scope4/1  "yFF"
  Saturation1/1 -> ThetaSet/1, Bus Creator/5  "yOut"
  Gain3/1 -> Bus Creator/4, Sum1/4, Scope4/3  "yD"
  Gain1/1 -> Bus Creator/2, Sum1/2, Scope4/2  "yP"
  Discrete-Time Integrator/1 -> Bus Creator/3, Sum1/3  "yI"
  Bus Creator/1 -> controllerOuts/1

== system subsystems/motor pressure controller/Voltage-VelocityCorrection ==
  OmegaDemand : Inport
  Gain : Gain  Gain=1/1100
  Gain1 : Gain  Gain=1/2
  Saturation : Saturate  UpperLimit=3  LowerLimit=-3
  Sign : Signum
  Sum : Sum  Inputs=|++
  Sum1 : Sum  Inputs=|+-
  DutyDemand : Outport
  wires:
  OmegaDemand/1 -> Saturation/1, Sum1/1
  Gain/1 -> Sum/2
  Sign/1 -> Gain1/1
  Gain1/1 -> Sum/1
  Sum/1 -> DutyDemand/1
  Saturation/1 -> Sum1/2
  Sum1/1 -> Sign/1, Gain/1

== system subsystems/motor velocity controller/clock ==
  reset : Inport
  Constant : Constant
  Constant1 : Constant  Value=0
  Delay : Delay  DelayLength=1  SampleTime=velocity_controller_Ts
  Sum : Sum  Inputs=|++
  Switch1 : Switch  Criteria=u2 > Threshold  SaturateOnIntegerOverflow=off  InputSameDT=off
  timer : Outport
  wires:
  Switch1/1 -> Delay/1, timer/1
  Constant/1 -> Sum/1
  Delay/1 -> Sum/2
  reset/1 -> Switch1/2
  Sum/1 -> Switch1/3
  Constant1/1 -> Switch1/1

== matlab function subsystems/P_nozzle lookup/P_nozzle lookup1 ==
  data: nozzlePressure output; manifold input; valveAngle input
function nozzlePressure  = fcn(manifold, valveAngle)

x = manifold;
y = valveAngle;


%% values with 0 motor angle correction and 0 manifold pressure corrections added
% added extra values to define the boundry conditions where pnozzle is zero
% if pmanifold is zero or theta motor is zero.
% fitted to a poly25 function instead of 
% p00 =  -12.4364367169073;
% p10 =  0.262880598460491;
% p01 =  -0.0274862894960315;
% p20 =  -0.00105126884821146;
% p11 =  0.00379948265766187;
% p02 =  9.57398900557826e-05;
% p21 =  4.61589989526699e-06;
% p12 =  -8.43503022917966e-06;
% p03 =  1.64107253476236e-07;
% p22 =  -6.22458938326231e-09;
% p13 =  7.94544459820422e-09;
% p04 =  -4.13354307582726e-10;
% p23 =  2.60630863468415e-12;
% p14 =  -2.64465586252337e-12;
% p05 =  1.92194586805639e-13;

p00 = -0.7981;
p10 = -0.1004;
p01 = 0.00818;
p20 = 0.0003445;
p11 = 0.004281;
p02 = -2.873e-05;
p30 = -1.178e-05;
p21 = -3.514e-06;
p12 = -5.16e-06;
p03 = 2.012e-08;
p40 = 9.558e-08;
p31 = 2.025e-08;
p22 = 1.016e-09;
p13 = 1.894e-09;
p50 = -1.955e-10;
p41 = -3.494e-11;
p32 = -1.12e-11;
p23 = 1.891e-12;


nozzlePressure = p00 + p10.*x + p01.*y + ...
    p20.*x.^2 + p11.*x.*y + p02*y.^2 + ...
    p30.*x.^3 + p21.*x.^2.*y + p12.*x.*y.^2 + p03.*y.^3 + ...
    p40.*x.^4 + p31.*x.^3.*y + p22.*x.^2.*y.^2 + p13.*x.*y.^3 + ...
    p50.*x.^5 + p41.*x.^4.*y + p32.*x.^3.*y.^2 + p23.*x.^2.*y.^3;
end

== matlab function subsystems/Valve_angle lookup/P_nozzle lookup1 ==
  data: valveAngle output double size=1 [0..1500]; manifold input double size=1; nozzle input double size=1; angle0 input
function valveAngle = valve_angle_lookup(manifold, nozzle, angle0)
x = manifold;
% y = nozzle;

%% values with 0 motor angle correction and 0 manifold pressure corrections added
% added extra values to define the boundry conditions where pnozzle is zero
% if pmanifold is zero or theta motor is zero.
% fitted to a poly25 function instead of 
% p00 =  -12.4364367169073;
% p10 =  0.262880598460491;
% p01 =  -0.0274862894960315;
% p20 =  -0.00105126884821146;
% p11 =  0.00379948265766187;
% p02 =  9.57398900557826e-05;
% p21 =  4.61589989526699e-06;
% p12 =  -8.43503022917966e-06;
% p03 =  1.64107253476236e-07;
% p22 =  -6.22458938326231e-09;
% p13 =  7.94544459820422e-09;
% p04 =  -4.13354307582726e-10;
% p23 =  2.60630863468415e-12;
% p14 =  -2.64465586252337e-12;
% p05 =  1.92194586805639e-13;

%% VOLKAN
p00 = -0.7981;
p10 = -0.1004;
p01 = 0.00818;
p20 = 0.0003445;
p11 = 0.004281;
p02 = -2.873e-05;
p30 = -1.178e-05;
p21 = -3.514e-06;
p12 = -5.16e-06;
p03 = 2.012e-08;
p40 = 9.558e-08;
p31 = 2.025e-08;
p22 = 1.016e-09;
p13 = 1.894e-09;
p50 = -1.955e-10;
p41 = -3.494e-11;
p32 = -1.12e-11;
p23 = 1.891e-12;


 % z = p00 + p10*x + p01*y + ...
 %        p20*x.^2 + p11*x.*y + p02*y.^2 + ...
 %        p30*x.^3 + p21*x.^2.*y + p12*x.*y.^2 + p03*y.^3 + ...
 %        p40*x.^4 + p31*x.^3.*y + p22*x.^2.*y.^2 + p13*x.*y.^3 + ...
 %        p50*x.^5 + p41*x.^4.*y + p32*x.^3.*y.^2 + p23*x.^2.*y.^3;

c0 = p00 + p10*x + p20*x.^2 + p30*x.^3 + p40*x.^4 + p50*x.^5;
c1 = p01 + p11*x + p21*x.^2 + p31*x.^3 + p41*x.^4; 
c2 = p02 + p12*x + p22*x.^2 + p32*x.^3;
c3 = p03 + p13*x + p23*x.^2;



polynomFunc = @(angle) c3 * angle^3 + c2 * angle^2 + c1 * angle + c0 - nozzle;
polynomFuncDer = @(angle) 3*c3 * angle^2 + 2*c2 * angle + c1;

% valveAngle = fzero(polynomFunc, 10);
% valveAngle = secant_method(polynomFunc, angle0, angle1, 1e-6, 20);
valveAngle = newton_raphson(polynomFunc, polynomFuncDer, angle0,0,1080,1e-6, 10);
valveAngle = min(valveAngle, 1000);
valveAngle = max(0, valveAngle);


end

== matlab function subsystems/motor_model/MATLAB Function ==
  data: v input; nu output; nu_d input; nu_s input; epsilon input; n input
function nu = fcn(v, nu_d, nu_s, epsilon, n)
%regularized friction block

alpha = sqrt(nu_s * (nu_s - nu_d));
num = - nu_d * v .* sqrt(v.^2 + epsilon ./ n^2) - 2 .* alpha ./ n .* v;
denum = v.^2 + 1 ./ n.^2;
nu = num ./ denum;


% nu = v;

== matlab function subsystems/Kalman Filter For Motor Position and Velocity/TPE_KALMAN_spd ==
  settings: updateMethod=DISCRETE  sampleTime=Ts
  data z settings: description=since it reads the encoder data its made uint32
  data: lambdaRQ input double size=1; velEst output double size=1; posEst output double size=1; qk output size=[2,1]; z input double size=1; qk input double size=[2,1]; Pk input double size=[2,2]; Ts parameter double size=1; Pk output size=[2,2]
function [ velEst, posEst, qk,Pk] =Kalman_X_Enc(lambdaRQ,z, qk, Pk, Ts)
%   200814 
%   --------
% INPUTS
%  z: measurement (1,1) %    [increment]
%   q1: previous state [2Nx1]
%   P1: previous error cov matrix [2Nx2N]
%   qk1: previous state [2x1]
%   Pk1: previous error cov matrix [2x2]
%   nSpindle : Spindle Speed [rpm]
%   IncrSec: increment per second
% PARAMETERS Periodic component
%   Ts      : Sampling time [ms]
%   Q :  process noise covariance matrix [2x2], tunable
%   R  :  measurement noise cov 1x1, tunable

%   R olcerdeki hataa,
%   Q modeldeki hata, Q kuculurse modele guvenir, smooth olur. Ama aynı isi
%   disaridan lambdaRQ carpani ile yapabilirsin.
R_Enc=0.08^2;
Q_Enc=[Ts^3/3, Ts^2/2; Ts^2/2, Ts]*(4/Ts)^2*1e-3;% <<<<<< BUNLA OYNA 1-4-10

%%  Remove the trend with kinematic Kalman Filter
Q=lambdaRQ*Q_Enc;
[qk,Pk] = Kalman_Kinematic(z, qk, Pk, R_Enc,Q,Ts);
velEst = qk(2);%[incr/sec]
posEst=qk(1);


end



function [q,P] = Kalman_Kinematic(z, q, P, R,Q,Ts)
%   First Eqn : Priori state est
PosPrior = q(1)+q(2)*Ts;
VelPrior =q(2);
%   Second Eqn : Priori cov matrix
dummy = P(2,1)+Ts*P(2,2);
P11 = P(1,1)+Ts*P(1,2) + Ts*dummy +Q(1,1);
P21 = dummy+Q(2,1);
P12 = P(1,2)+Ts*P(2,2)+Q(1,2);
P22 = P(2,2)+Q(2,2);

%   Kalman Gain
dummy = 1/(P11+R);
K1= P11*dummy;
K2= P21*dummy; % No need since there is no vel estimate

% State estimate
dummy=z-PosPrior;
q = [PosPrior + K1*dummy;...
    VelPrior+K2*dummy];

%   Covariance Matrix
P=[P11-K1*P11, P12-K1*P12;...
    P21-K2*P11, P22-K2*P12];
end

== matlab function subsystems/Valve_angle lookup/P_nozzle lookup ==
  data: ysol output double size=1 [0..1500]; x_fixed input double size=1; z_target input double size=1
function ysol = inverse_surface_fit_func(x_fixed, z_target)
    % x_fixed --> manifold basıncı
    % z_target --> lüle basınç isteri
    % ysol --> motor açısı çıktısı
    
    p00 = -5.366;
    p10 = -0.00758;
    p01 = 0.02057;
    p20 = -0.0007234;
    p11 = 0.001413;
    p02 = -1.563e-05;
    p30 = 6.092e-06;
    p21 = -1.277e-06;
    p12 = -7.057e-07;
    p40 = -1.199e-08;
    p31 = 1.98e-09;
    p22 = 7.056e-10;

    % Polinom katsayıları (y polinom)
    c2 = p02 + p12*x_fixed + p22*x_fixed^2;
    c1 = p01 + p11*x_fixed + p21*x_fixed^2 + p31*x_fixed^3;
    c0 = p00 + p10*x_fixed + p20*x_fixed^2 + p30*x_fixed^3 + p40*x_fixed^4 - z_target;

    d = c1^2-4*c2*c0;
    
    if d < 0
        ysol = -c1/(2*c2);
    else
        ysol = (-c1 + sqrt(d))/(2*c2);
    end    
    
end

== matlab function subsystems/P_nozzle lookup/P_nozzle lookup ==
  data: z output; x input; y input
function z = surface_fit_func(x,y)
    % x --> manifold basıncı
    % y --> motor açısı
    % z --> nozzle basıncı
    
    p00 = -5.366;
    p10 = -0.00758;
    p01 = 0.02057;
    p20 = -0.0007234;
    p11 = 0.001413;
    p02 = -1.563e-05;
    p30 = 6.092e-06;
    p21 = -1.277e-06;
    p12 = -7.057e-07;
    p40 = -1.199e-08;
    p31 = 1.98e-09;
    p22 = 7.056e-10;

    z = p00 + p10*x + p01*y + ...
        p20*x.^2 + p11*x.*y + p02*y.^2 + ...
        p30*x.^3 + p21*x.^2.*y + p12*x.*y.^2 + ...
        p40*x.^4 + p31*x.^3.*y + p22*x.^2.*y.^2;
end

== matlab function subsystems/motor_model_with_bumpstops_and_regularized_stribeck_friction/MATLAB Function ==
  data: v input; nu output; nu_d input; nu_s input; epsilon input; n input
function nu = fcn(v, nu_d, nu_s, epsilon, n)
%regularized friction block

alpha = sqrt(nu_s * (nu_s - nu_d));
num = - nu_d * v .* sqrt(v.^2 + epsilon ./ n^2) - 2 .* alpha ./ n .* v;
denum = v.^2 + 1 ./ n.^2;
nu = num ./ denum;


% nu = v;

== matlab function subsystems/MATLAB Function ==
  data: F output; t input
function F = osmansForceFunction(t)
    F1 = @(t) 1.5299.*10.^4.*t.^3 - 1.1012.*10.^04.*t.^2 + 2.6848.*10.^3.*t -57.7349;
    F2 = @(t) 6.7228.*10.^3.*t.^3 - 6.0413.*10.^03.*t.^2 + 1.7113.*10.^3.*t +6.7577;
    F3 = @(t) 151.2319.*exp(-0.9536.*t)+49.8264.*exp(-0.3823.*t);
    
    if t < 0.0230
        F = 0;  
    elseif t < 0.2070
        F = F1(t);
    elseif  t < 0.2810
        F = F2(t);
    elseif t >= 0.2810
        F = F3(t);
    else 
        F = 0;
    end
end

== matlab function subsystems/Kalman Filter For Platform Position and Velocity/TPE_KALMAN_spd ==
  settings: updateMethod=DISCRETE  sampleTime=Ts
  data z settings: description=since it reads the encoder data its made uint32
  data: lambdaRQ input double size=1; velEst output double size=1; posEst output double size=1; qk output size=[2,1]; z input double size=1; qk input double size=[2,1]; Pk input double size=[2,2]; Ts parameter double size=1; Pk output size=[2,2]
function [ velEst, posEst, qk,Pk] =Kalman_X_Enc(lambdaRQ,z, qk, Pk, Ts)
%   200814 
%   --------
% INPUTS
%  z: measurement (1,1) %    [increment]
%   q1: previous state [2Nx1]
%   P1: previous error cov matrix [2Nx2N]
%   qk1: previous state [2x1]
%   Pk1: previous error cov matrix [2x2]
%   nSpindle : Spindle Speed [rpm]
%   IncrSec: increment per second
% PARAMETERS Periodic component
%   Ts      : Sampling time [ms]
%   Q :  process noise covariance matrix [2x2], tunable
%   R  :  measurement noise cov 1x1, tunable

%   R olcerdeki hataa,
%   Q modeldeki hata, Q kuculurse modele guvenir, smooth olur. Ama aynı isi
%   disaridan lambdaRQ carpani ile yapabilirsin.
R_Enc=0.01^2;
Q_Enc=[Ts^3/3, Ts^2/2; Ts^2/2, Ts]*(4/Ts)^2*1e-3;% <<<<<< BUNLA OYNA 1-4-10

%%  Remove the trend with kinematic Kalman Filter
Q=lambdaRQ*Q_Enc;
[qk,Pk] = Kalman_Kinematic(z, qk, Pk, R_Enc,Q,Ts);
velEst = qk(2);%[incr/sec]
posEst=qk(1);


end



function [q,P] = Kalman_Kinematic(z, q, P, R,Q,Ts)
%   First Eqn : Priori state est
PosPrior = q(1)+q(2)*Ts;
VelPrior =q(2);
%   Second Eqn : Priori cov matrix
dummy = P(2,1)+Ts*P(2,2);
P11 = P(1,1)+Ts*P(1,2) + Ts*dummy +Q(1,1);
P21 = dummy+Q(2,1);
P12 = P(1,2)+Ts*P(2,2)+Q(1,2);
P22 = P(2,2)+Q(2,2);

%   Kalman Gain
dummy = 1/(P11+R);
K1= P11*dummy;
K2= P21*dummy; % No need since there is no vel estimate

% State estimate
dummy=z-PosPrior;
q = [PosPrior + K1*dummy;...
    VelPrior+K2*dummy];

%   Covariance Matrix
P=[P11-K1*P11, P12-K1*P12;...
    P21-K2*P11, P22-K2*P12];
end

== matlab function subsystems/Kalman Filter For Platform Position and Velocity/MATLAB Function ==
  data: u1 input; y output
function y = fcn(u1)

y = [u1; 0.0];

== matlab function subsystems/euler 2 quaternion/MATLAB Function ==
  data: u1 input size=1; y1 output size=1; u2 input size=1; u3 input; y2 output size=1; y3 output size=1; y4 output size=1
function [y1, y2, y3, y4] = fcn(u1, u2, u3)
    q = eul2quat([u1 u2 u3]);
    y1 = q(1);
    y2 = q(2);
    y3 = q(3);
    y4 = q(4);
end
